simulink model "test_plant"  (R2018b)
settings: Solver=FixedStepAuto  StartTime=0.0  StopTime=inf  FixedStep=0.00001  RelTol=1e-3
values from neighbouring files (symbols this model uses):
  K = -K    (= -0.383)    [LQG_control_design.m]    (also in LQR_control_design.m = -(1/R).*B'*Sinf; myLQR.m = -(1/R).*B'*Sinf; myREF.m = [Kw Ki])
libraries: fl_lib x5, nesl_utility x5, elec_lib x1
settings Model: Creator=angel  LastModifiedBy=angel
settings SolverCC: ZeroCrossAlgorithm=Adaptive
settings DebuggingCC: IgnoredZcDiagnostic=none

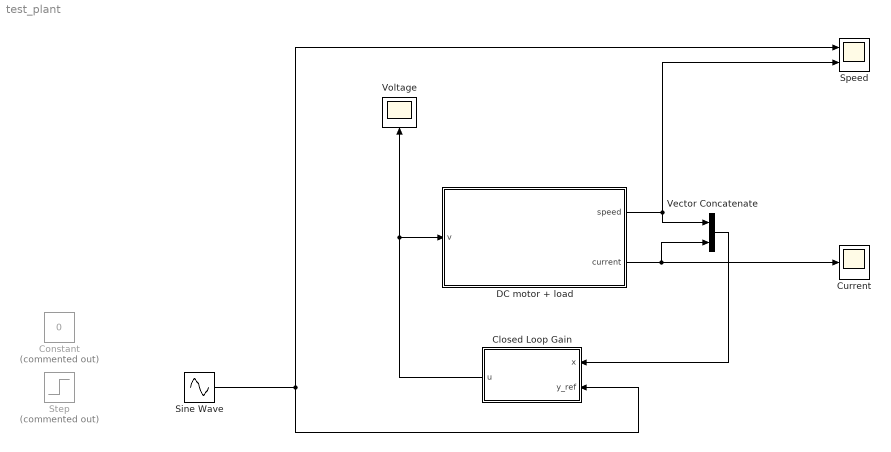
== system test_plant ==
  Closed Loop Gain : Subsystem
  Constant : Constant  Commented=on  Value=0
  Current : Scope
  DC motor + load : Subsystem  ClipboardFcn=run('init_throttle.m')
  Sine Wave : Sin  Amplitude=5  SampleTime=0
  Speed : Scope  NumInputPorts=2
  Step : Step  Commented=on  Time=5  SampleTime=0
  Vector Concatenate : Concatenate
  Voltage : Scope
  wires:
  DC motor + load/1(speed) -> Vector Concatenate/1, Speed/2
  DC motor + load/2(current) -> Current/1, Vector Concatenate/2
  Sine Wave/1 -> Closed Loop Gain/2(y_ref), Speed/1
  Closed Loop Gain/1(u) -> DC motor + load/1(v), Voltage/1
  Vector Concatenate/1 -> Closed Loop Gain/1(x)

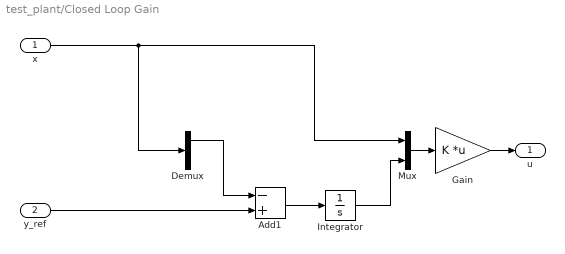
== system test_plant/Closed Loop Gain ==
  x : Inport
  y_ref : Inport  Port=2
  Add1 : Sum  Inputs=-+
  Demux : Demux  Outputs=2
  Gain : Gain  Gain=K  Multiplication=Matrix(K*u) (u vector)
  Integrator : Integrator
  Mux : Mux  Inputs=2
  u : Outport
  wires:
  x/1 -> Demux/1, Mux/1
  Add1/1 -> Integrator/1
  Integrator/1 -> Mux/2
  Gain/1 -> u/1
  y_ref/1 -> Add1/2
  Demux/1 -> Add1/1
  Mux/1 -> Gain/1

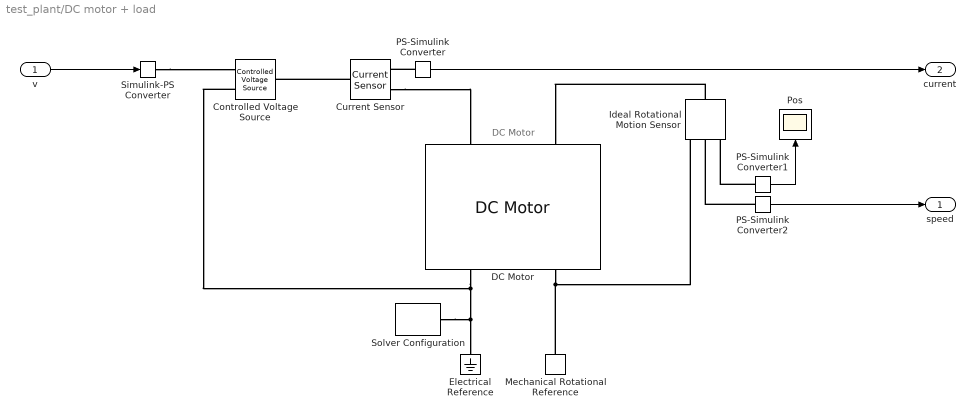
== system test_plant/DC motor + load ==
  note: DC Motor
  v : Inport
  Controlled Voltage Source : fl_lib/Electrical/Electrical Sources/Controlled Voltage Source
  Current Sensor : fl_lib/Electrical/Electrical Sensors/Current Sensor
  DC Motor : elec_lib/Actuators & Drivers/Rotational Actuators/DC Motor  parameterization=1  Ra=1.15 Ohm  La=1.5 mH  emf_or_torque=1  Kv=0.383 V/(rad/s)  Ki=6.876e-4 N*m/A  T_stall=0.24e-3 N*m  w_max=19100 rpm  w_rated=15000 rpm  P_rated=0.08 W  V_rated=1.5 V  J=0.021 kg*m^2  lam_param=1  lam=0.087 N*m/(rad/s)  i_noload=0 A  V_i_noload=1.5 V  speed0=10 rad/s  alpha=3.93e-3 1/K  Tmeas=25 degC  thermal_mass=100 J/K  initial_temperature=25 degC
  Electrical Reference : fl_lib/Electrical/Electrical Elements/Electrical Reference
  Ideal Rotational Motion Sensor : fl_lib/Mechanical/Mechanical Sensors/Ideal Rotational Motion Sensor  offset=0 rad
  Mechanical Rotational Reference : fl_lib/Mechanical/Rotational Elements/Mechanical Rotational Reference
  PS-Simulink Converter : nesl_utility/PS-Simulink Converter  PhysicalDomain=network_engine_domain  SubClassName=ps_output  LeftPortType=input  RightPortType=output  PseudoPeriodic=off  Frequencies=[]  Unit=A  AffineConversion=off
  PS-Simulink Converter1 : nesl_utility/PS-Simulink Converter  PhysicalDomain=network_engine_domain  SubClassName=ps_output  LeftPortType=input  RightPortType=output  PseudoPeriodic=off  Frequencies=[]  Unit=rad  AffineConversion=off
  PS-Simulink Converter2 : nesl_utility/PS-Simulink Converter  PhysicalDomain=network_engine_domain  SubClassName=ps_output  LeftPortType=input  RightPortType=output  PseudoPeriodic=off  Frequencies=[]  Unit=rad/s  AffineConversion=off
  Pos : Scope
  Simulink-PS Converter : nesl_utility/Simulink-PS Converter  PhysicalDomain=network_engine_domain  SubClassName=ps_input  LeftPortType=input  RightPortType=output  PseudoPeriodic=off  Frequencies=[]  NoiseDistribution=none  NoiseParameters=[]  Unit=V  AffineConversion=off  FilteringAndDerivatives=provide  SimscapeFilterOrder=1  InputFilterTimeConstant=0.001  UdotUserProvided=0
  Solver Configuration : nesl_utility/Solver Configuration  PhysicalDomain=network_engine_domain  SubClassName=solver  LeftPortType=input  RightPortType=generic  Tones=[]  Harmonics=[]  SimulateNoise=off  Profile=off  UseLocalSampling=off  EnableSwitchedLinearOptims=on  FrequencyDomain=off  UseCCode=off  RelTol=0.001  AbsTol=1e-06  MinStep=1e-09  ToWorkspace=off  RevertToSquareIcSolve=off  NumHomotopyIterations=100  PhasorMode=off  PhasorModeNumHarmonics=1  DoDC=off  ResidualTolerance=1e-09  UseLocalSolver=off  LocalSolverChoice=NE_BACKWARD_EULER_ADVANCER  LocalSolverSampleTime=0.001  DoFixedCost=off  MaxNonlinIter=3  MaxModeIter=2  LinearAlgebra=auto  EquationFormulation=NE_TIME_EF  DelaysMemoryBudget=1024  AutomaticFiltering=on  FilteringTimeConstant=0.001  PartitionStorageMethod=AS_NEEDED  PartitionMemoryBudget=1024
  speed : Outport
  current : Outport  Port=2
  wires:
  PS-Simulink Converter2/1 -> speed/1
  v/1 -> Simulink-PS Converter/1
  PS-Simulink Converter1/1 -> Pos/1
  PS-Simulink Converter/1 -> current/1
  connections:
  Ideal Rotational Motion Sensor/LConn1 -- DC Motor/LConn2
  DC Motor/RConn2 -- Ideal Rotational Motion Sensor/RConn1 -- Mechanical Rotational Reference/LConn1
  DC Motor/RConn1 -- Controlled Voltage Source/RConn2 -- Solver Configuration/RConn1 -- Electrical Reference/LConn1
  Current Sensor/RConn2 -- DC Motor/LConn1
  PS-Simulink Converter/LConn1 -- Current Sensor/RConn1
  Simulink-PS Converter/RConn1 -- Controlled Voltage Source/RConn1
  PS-Simulink Converter1/LConn1 -- Ideal Rotational Motion Sensor/RConn3
  PS-Simulink Converter2/LConn1 -- Ideal Rotational Motion Sensor/RConn2
  Current Sensor/LConn1 -- Controlled Voltage Source/LConn1
